simulink model "Active_Suspension_1_Simulink"  (R2023b)
settings: Solver=VariableStepAuto  StartTime=0.0  StopTime=100.0  MaxStep=1e-4  RelTol=1e-3
values from neighbouring files (symbols this model uses):
  cc = 30    [Extras.m]
  cu_robust = 10    [Extras.m]
undefined symbols (not defined in the file or in its folder): kc, kw, mc, mw
settings Model: Creator=hkurt  LastModifiedBy=hkurt

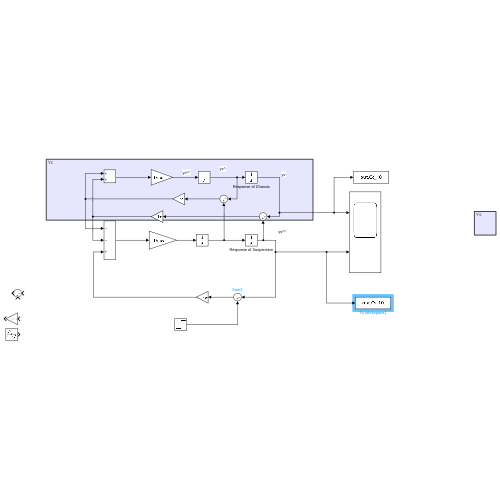
[thumbnail: Simulink's stored preview of the top-level diagram]
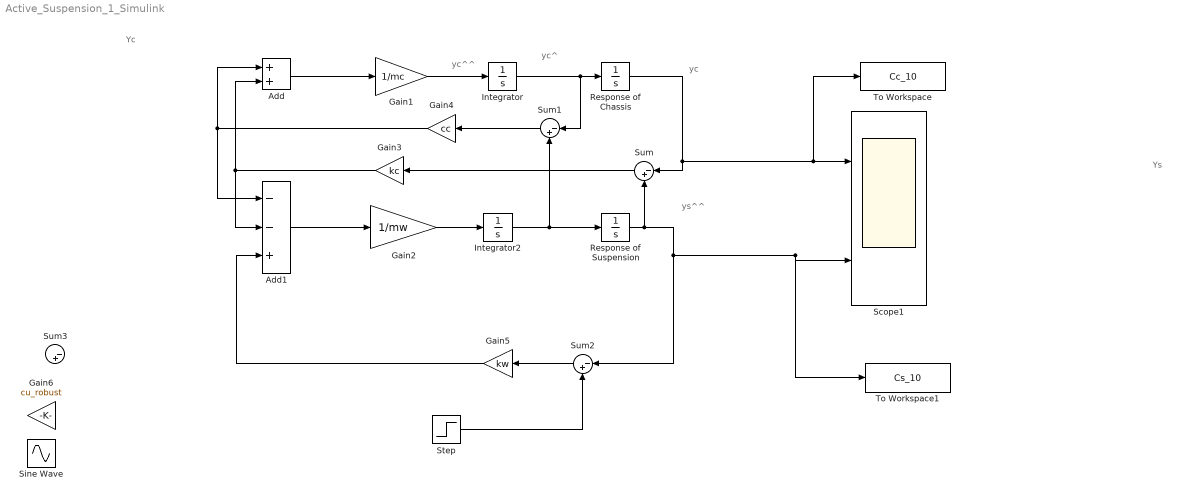
== system Active_Suspension_1_Simulink ==
  note: yc
  note: Ys
  note: Yc
  note: ys^^
  note: yc^
  note: yc^^
  Add : Sum
  Add1 : Sum  Inputs=--+
  Gain1 : Gain  Gain=1/mc
  Gain2 : Gain  Gain=1/mw
  Gain3 : Gain  Gain=kc
  Gain4 : Gain  Gain=cc
  Gain5 : Gain  Gain=kw
  Gain6 : Gain  Gain=cu_robust
  Integrator : Integrator
  Integrator2 : Integrator
  Response of Chassis : Integrator
  Response of Suspension : Integrator
  Scope1 : Scope  NumInputPorts=2
  Sine Wave : Sin  Amplitude=30  Frequency=5  SampleTime=0
  Step : Step  After=20  SampleTime=0
  Sum{,1..3} (4 alike) : Sum  Inputs=|-+
  To Workspace : ToWorkspace  VariableName=Cc_10  SaveFormat=Timeseries  SampleTime=-1
  To Workspace1 : ToWorkspace  VariableName=Cs_10  SaveFormat=Timeseries  SampleTime=-1
  wires:
  Gain1/1 -> Integrator/1
  Integrator/1 -> Sum1/1, Response of Chassis/1
  Add/1 -> Gain1/1
  Add1/1 -> Gain2/1
  Gain2/1 -> Integrator2/1
  Integrator2/1 -> Sum1/2, Response of Suspension/1
  Response of Chassis/1 -> Sum/1, To Workspace/1, Scope1/1
  Response of Suspension/1 -> Sum/2, Sum2/1, To Workspace1/1, Scope1/2
  Sum/1 -> Gain3/1
  Sum1/1 -> Gain4/1
  Sum2/1 -> Gain5/1
  Gain5/1 -> Add1/3
  Gain3/1 -> Add1/2, Add/2
  Gain4/1 -> Add1/1, Add/1
  Step/1 -> Sum2/2
